simulink model "bloques_tp_compatible"  (R2023a)
settings: Solver=VariableStepAuto  StartTime=0.0  StopTime=10.0  RelTol=1e-3
libraries: commchan3 x1
settings Model: Creator=mechi  LastModifiedBy=mechi

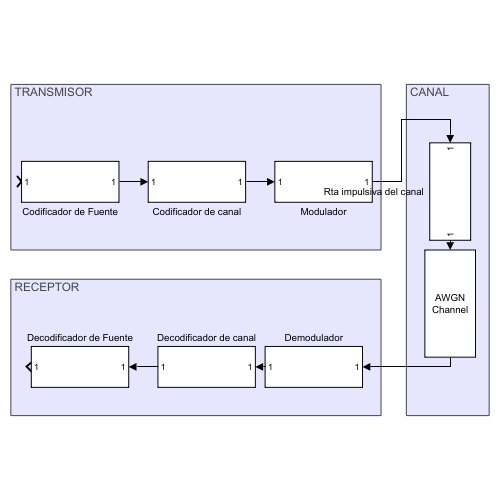
[thumbnail: Simulink's stored preview of the top-level diagram]
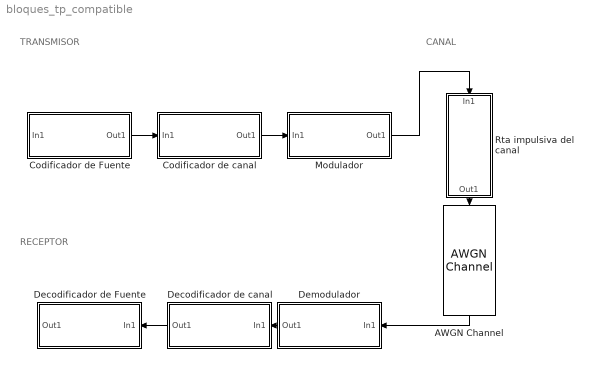
== system bloques_tp_compatible ==
  note: RECEPTOR
  note: CANAL
  note: TRANSMISOR
  AWGN Channel : commchan3/AWGN Channel  LegacyMode=off  NoiseMethod="Signal to noise ratio  (SNR)"  noiseMode="Signal to noise ratio  (SNR)"  EbNo=10  EsNo=10  SNR=10  BitsPerSymbol=1  SignalPower=1  SamplesPerSymbol=1  SymbolPeriod=1  VarianceSource=Parameter  Variance=1  RandomStream=Global stream  Seed=67  SimulateUsing=Code generation
  Codificador de Fuente : Subsystem
  Codificador de canal : Subsystem
  Decodificador de Fuente : Subsystem
  Decodificador de canal : Subsystem
  Demodulador : Subsystem
  Modulador : Subsystem
  Rta impulsiva del canal : Subsystem
  wires:
  Codificador de Fuente/1(Out1) -> Codificador de canal/1(In1)
  Codificador de canal/1(Out1) -> Modulador/1(In1)
  Modulador/1(Out1) -> Rta impulsiva del canal/1(In1)
  Demodulador/1(Out1) -> Decodificador de canal/1(In1)
  Decodificador de canal/1(Out1) -> Decodificador de Fuente/1(In1)
  Rta impulsiva del canal/1(Out1) -> AWGN Channel/1
  AWGN Channel/1 -> Demodulador/1(In1)

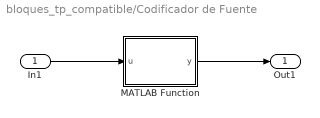
== system bloques_tp_compatible/Codificador de Fuente ==
  In1 : Inport
  MATLAB Function : MATLAB Function  TreatAsAtomicUnit=on
  Out1 : Outport
  wires:
  In1/1 -> MATLAB Function/1(u)
  MATLAB Function/1(y) -> Out1/1

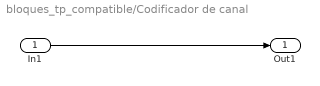
== system bloques_tp_compatible/Codificador de canal ==
  In1 : Inport
  Out1 : Outport
  wires:
  In1/1 -> Out1/1

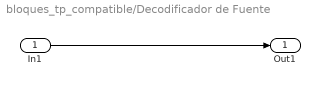
== system bloques_tp_compatible/Decodificador de Fuente ==
  In1 : Inport
  Out1 : Outport
  wires:
  In1/1 -> Out1/1

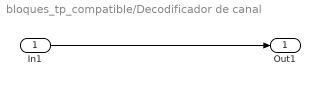
== system bloques_tp_compatible/Decodificador de canal ==
  In1 : Inport
  Out1 : Outport
  wires:
  In1/1 -> Out1/1

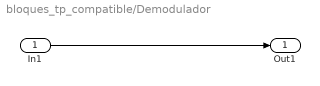
== system bloques_tp_compatible/Demodulador ==
  In1 : Inport
  Out1 : Outport
  wires:
  In1/1 -> Out1/1

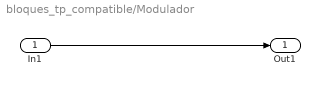
== system bloques_tp_compatible/Modulador ==
  In1 : Inport
  Out1 : Outport
  wires:
  In1/1 -> Out1/1

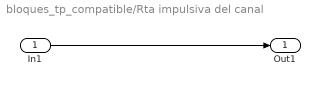
== system bloques_tp_compatible/Rta impulsiva del canal ==
  In1 : Inport
  Out1 : Outport
  wires:
  In1/1 -> Out1/1

== matlab function bloques_tp_compatible/Codificador de Fuente/MATLAB Function ==
  data: u input; y output
function y = fcn(u)

%abrir_archivo(ruta);
%char[], proba[] lectura_archivo(archivo);
%float calcular_entropia_fuente(proba[]);
%dict huffmandict();
%float longitud_minima(dict);
%float longitud_promedio(dict);
%palabras[] codificar(archivo, dict);

y = u;
